simulink model "Traffic_Flow_simulation"  (R2021a)
settings: Solver=FixedStepAuto  StartTime=0.0  StopTime=inf  RelTol=1e-4
model workspace (MAT data in the model file):
  RefVel = 0.1
values from neighbouring files (symbols this model uses):
  NPC_waypoints = NPC_waypoints(:,1:2)    [setup.m]    (also in waypoint_genearator.m)
  waypoints = waypoints(:,1:2)    [setup.m]    (also in waypoint_genearator.m)
libraries: visionsinks x4, drivingvehiclecontroller x1, robotalgslib x1
(part 2 of 2)

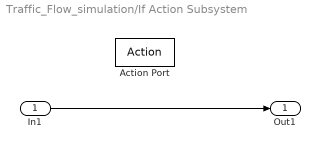
== system Traffic_Flow_simulation/If Action Subsystem ==
  In1 : Inport
  Action Port : ActionPort  ActionPortLabel=if(u1 > 0)
  Out1 : Outport
  wires:
  In1/1 -> Out1/1

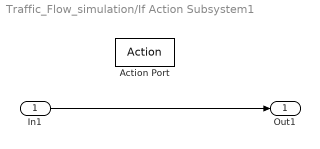
== system Traffic_Flow_simulation/If Action Subsystem1 ==
  In1 : Inport
  Action Port : ActionPort  ActionPortLabel=if(u1 > 0)
  Out1 : Outport
  wires:
  In1/1 -> Out1/1

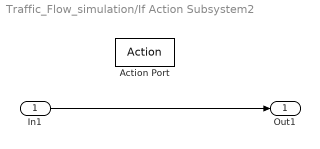
== system Traffic_Flow_simulation/If Action Subsystem2 ==
  In1 : Inport
  Action Port : ActionPort  ActionPortLabel=if(u1 > 0)
  Out1 : Outport
  wires:
  In1/1 -> Out1/1

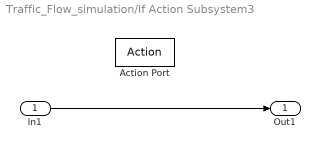
== system Traffic_Flow_simulation/If Action Subsystem3 ==
  In1 : Inport
  Action Port : ActionPort  ActionPortLabel=if(u1 > 0)
  Out1 : Outport
  wires:
  In1/1 -> Out1/1

== matlab function Traffic_Flow_simulation/LEAD ASSIGMENT ==
  data: traffic_vehicle_information input; l1 output; l2 output; l3 output; ego_vehicle_information input
function [l1,l2,l3]= fcn(traffic_vehicle_information,ego_vehicle_information)
    

    if ego_vehicle_information(2) > 5
        vehicle_information = [traffic_vehicle_information,ego_vehicle_information];
        vehicle_information = reshape(vehicle_information,4,length(vehicle_information)/4);
    else
        vehicle_information = reshape(traffic_vehicle_information,4,length(traffic_vehicle_information)/4);
    end

    x = vehicle_information(1,:);
    v = vehicle_information(4,:);
    
    output = zeros(length(x),3);
    output(:,1) = (x == min(x));

    lead_pos_id = zeros(1,length(x));
    for i = 1:length(x)
        if output(i,1)
            lead_pos_id(i) = i;
        else
            y = (x(i)-x);
            y(y<=0) = NaN;
            [~,ind] = min(y);
            lead_pos_id(i) = ind;
        end
    end

    output(:,2) = x(lead_pos_id);
    output(:,3) = v(lead_pos_id);
    
    
    l1 = output(1,1:3);
    l2 = output(2,1:3);
    l3 = output(3,1:3); 
end

== matlab function Traffic_Flow_simulation/MATLAB Function ==
  data: pos input; y output; merging_area input; radius input
function y = fcn(pos,merging_area,radius)

    y = (sqrt( (pos(1)-merging_area(1))^2 + (pos(2)-merging_area(2))^2 ) < radius);

end

== matlab function Traffic_Flow_simulation/MATLAB Function1 ==
  data: fg input; y output; bg input; b_threshold input; f_threshold input
function y = fcn(fg,bg,b_threshold,f_threshold)

y = (bg < b_threshold) || (fg < f_threshold );
